simulink model "even_test"  (R2021a)
settings: Solver=VariableStepAuto  StartTime=0.0  StopTime=1  RelTol=1e-3
settings Model: Creator=DELL  LastModifiedBy=DELL

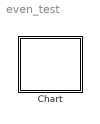
== system even_test ==
  Chart : Stateflow chart  TreatAsAtomicUnit=on

== stateflow chart even_test/Chart ==
  state a [parallel]
    en:
    sfdbg('a.en')
    du:
    sfdbg('a.du')
    send(disarm,c.disarm1)
    ex:
    sfdbg('a.ex')
    settings: executionOrder=1
  state b [parallel]
    en:
    sfdbg('b.en')
    du:
    sfdbg('b.du')
    ex:
    sfdbg('b.ex')
    settings: executionOrder=2
  state c [parallel]
    en:
    sfdbg('c.en')
    du:
    sfdbg('c.du')
    ex:
    sfdbg('c.ex')
    settings: executionOrder=3
    state arm1
      en:
      sfdbg('arm.en')
      du:
      sfdbg('arm.du')
      ex:
      sfdbg('arm.ex')
    state disarm1
      en:
      sfdbg('dis.en')
      du:
      sfdbg('dis.du')
      ex:
      sfdbg('dis.ex')
    disarm1 -> arm1 : arm
    arm1 -> disarm1 : disarm
    (default) -> disarm1
  events: disarm local FUNCTION_CALL_EVENT; arm local FUNCTION_CALL_EVENT
